simulink model "Project2"  (R2024b)
settings: Solver=VariableStepAuto  StartTime=0.0  StopTime=4  RelTol=1e-3
values from neighbouring files (symbols this model uses):
  Cl = 2000e-6    (= 0.002)    [ScriptFile.m]
  ka = Vdcref / 2    (= 350)    [ScriptFile.m]
  kii = 2 * pi * fbwi * Rl / ka    (= 0.0538558740615)    [ScriptFile.m]
  kiw = Vq / Vdcref    [ScriptFile.m]
  kpi = 2 * pi * fbwi * Ll / ka    (= 0.134639685154)    [ScriptFile.m]
  kpw = 2 * Cl / (kiw * a_l * tau1l)    [ScriptFile.m]
  Ll = 5e-3    (= 0.005)    [ScriptFile.m]
  Rbat = (Vdcref / Pdc) * (Vbat - Vdcref)    (= 7)    [ScriptFile.m]
  Rl = 0.002    [ScriptFile.m]
  tau_fl = 1 / (2 * pi * 100)    (= 0.00159154943092)    [ScriptFile.m]
  Vdcref = 700    [ScriptFile.m]
libraries: spsVoltageMeasurementLib x7, spsIGBTDiodeLib x6, spsSeriesRLCBranchLib x4, spsCurrentMeasurementLib x3, simulink x3, spsThreePhaseSeriesRLCBranchLib x2, spsBreakerLib x1, spsControlledVoltageSourceLib x1, spsTriangleGeneratorLib x1, spsThreePhaseBreakerLib x1, spsThreePhaseSourceLib x1, sps_lib x1
settings Model: Creator=SSP Family  LastModifiedBy=PREKSHA

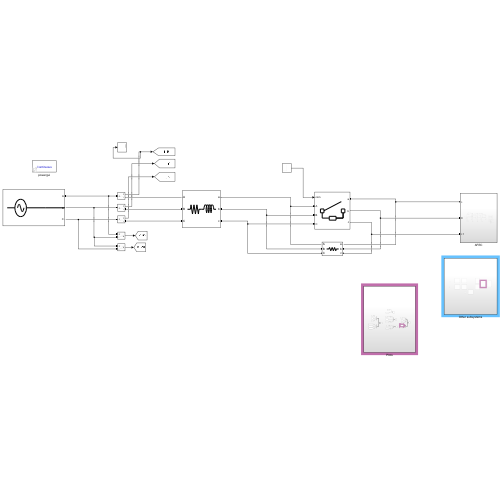
[thumbnail: Simulink's stored preview of the top-level diagram]
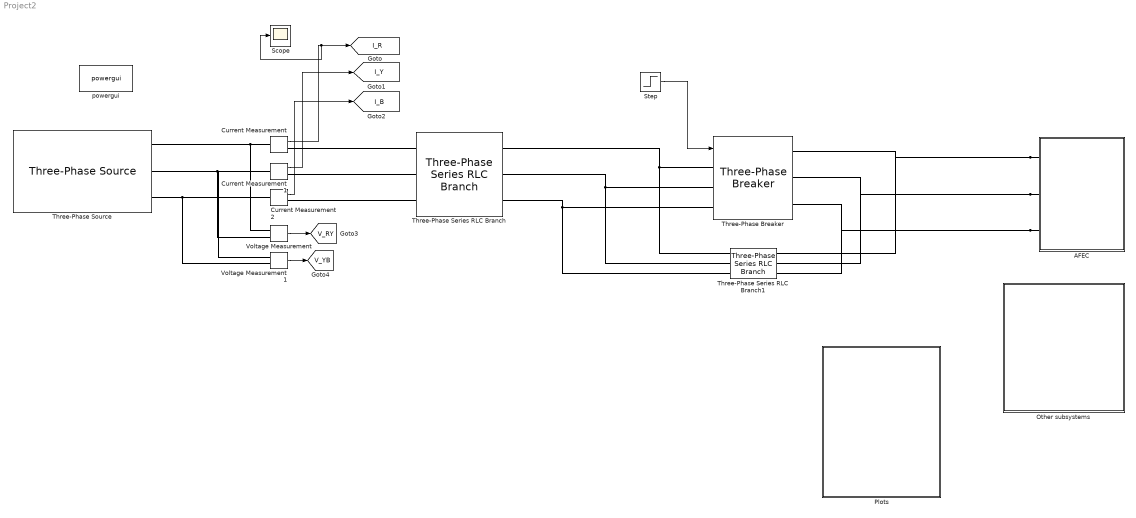
== system Project2 ==
  AFEC : Subsystem
  Current Measurement : spsCurrentMeasurementLib/Current Measurement  PhasorSimulation=off  OutputType=Complex  PSBequivalent=0
  Current Measurement1 : spsCurrentMeasurementLib/Current Measurement  PhasorSimulation=off  OutputType=Complex  PSBequivalent=0
  Current Measurement2 : spsCurrentMeasurementLib/Current Measurement  PhasorSimulation=off  OutputType=Complex  PSBequivalent=0
  Other subsystems : Subsystem
  Plots : Subsystem
  Scope : Scope
  Step : Step  Time=0.4  SampleTime=0
  Three-Phase Series RLC Branch : spsThreePhaseSeriesRLCBranchLib/Three-Phase Series RLC Branch  LConnTagsString=A|B|C  RConnTagsString=A|B|C  BranchType=RL  Resistance=Rl  Inductance=Ll  Capacitance=1e-6  Measurements=None
  Three-Phase Series RLC Branch1 : spsThreePhaseSeriesRLCBranchLib/Three-Phase Series RLC Branch  LConnTagsString=A|B|C  RConnTagsString=A|B|C  BranchType=R  Resistance=100  Inductance=1e-3  Capacitance=1e-6  Measurements=None
  Three-Phase Breaker : spsThreePhaseBreakerLib/Three-Phase Breaker  InitialState=open  SwitchA=on  SwitchB=on  SwitchC=on  SwitchTimes="[1/60  5/60]"  External=on  BreakerResistance=0.01  SnubberResistance=1e6  SnubberCapacitance=inf  Measurements=None
  Three-Phase Source : spsThreePhaseSourceLib/Three-Phase Source  InternalConnection=Y  VoltagePhases=off  Voltage=400/sqrt(3)  PhaseAngle=0  Voltage_phases=[25e3 25e3 25e3]/sqrt(3)  PhaseAngles_phases=[0 -120 +120]  Frequency=50  NonIdealSource=off  SpecifyImpedance=off  Resistance=0  Inductance=0  ShortCircuitLevel=100e6  BaseVoltage=25e3  XRratio=7  BusType=swing  Pref=10e3  Qref=0  Prefabc=[10e3, 10e3, 10e3]  Qrefabc=[0, 0, 0]  Qmin=-inf  Qmax=inf
  Voltage Measurement : spsVoltageMeasurementLib/Voltage Measurement  PhasorSimulation=off  OutputType=Complex  PSBequivalent=0
  Voltage Measurement1 : spsVoltageMeasurementLib/Voltage Measurement  PhasorSimulation=off  OutputType=Complex  PSBequivalent=0
  powergui : sps_lib/powergui  Priority=1  SimulationMode=Continuous  SampleTime=50e-6  frequency=60  Iterations=50  frequencyindice=50  Pbase=100e6  ErrMax=1e-4  UnitsV=kV  UnitsW=MW  buscounter=0  FunctionMessages=off  echomessages=off  EnableUseOfTLC=off  CurrentSourceSwitches=off  DisableSnubberDevices=off  DisableRonSwitches=off  DisableVfSwitches=off  DisplayEquations=off  AutomaticDiscreteSolvers=off  SolverType=Tustin/Backward Euler (TBE)  Interpol=off  ExternalGateDelay=off  methode=off  Ts=100  x0status=blocks  SPID=on  SwTol=0  HookPort=off  NonlinearTolerance=1e-4  nMaxIteration=100  ContinueOnMaxIteration=off  RestoreLinks=warning  ResistiveCurrentMeasurement=off  Frange=[0:2:500]  Ylog=off  Xlog=on  ShowGrid=off  save=off  variable=ZData  structure=0  ZoomFFT=off  StartTime=0.0  cycles=1  DisplayStyle=1  fundamental=60  FreqAxis=off  MaxFrequency=1000  frequencyindicesteady=1  RmsSteady=1  display=off
  tag scope: I_B=global, I_R=global, I_Y=global, V_RY=global, V_YB=global
  wires:
  Voltage Measurement/1 -> [V_RY]
  Voltage Measurement1/1 -> [V_YB]
  Step/1 -> Three-Phase Breaker/1
  Current Measurement/1 -> Scope/1, [I_R]
  Current Measurement1/1 -> [I_Y]
  Current Measurement2/1 -> [I_B]
  connections:
  Current Measurement/LConn1 -- Voltage Measurement/LConn1 -- Three-Phase Source/RConn1
  Current Measurement1/LConn1 -- Voltage Measurement1/LConn1 -- Voltage Measurement/LConn2 -- Three-Phase Source/RConn2
  Three-Phase Source/RConn3 -- Voltage Measurement1/LConn2 -- Current Measurement2/LConn1
  Current Measurement/RConn1 -- Three-Phase Series RLC Branch/LConn1
  Current Measurement1/RConn1 -- Three-Phase Series RLC Branch/LConn2
  Current Measurement2/RConn1 -- Three-Phase Series RLC Branch/LConn3
  Three-Phase Series RLC Branch1/LConn2 -- Three-Phase Series RLC Branch/RConn2 -- Three-Phase Breaker/LConn2
  Three-Phase Series RLC Branch1/LConn1 -- Three-Phase Series RLC Branch/RConn1 -- Three-Phase Breaker/LConn1
  AFEC/LConn1 -- Three-Phase Breaker/RConn1 -- Three-Phase Series RLC Branch1/RConn1
  Three-Phase Series RLC Branch1/LConn3 -- Three-Phase Series RLC Branch/RConn3 -- Three-Phase Breaker/LConn3
  AFEC/LConn3 -- Three-Phase Breaker/RConn3 -- Three-Phase Series RLC Branch1/RConn3
  AFEC/LConn2 -- Three-Phase Breaker/RConn2 -- Three-Phase Series RLC Branch1/RConn2

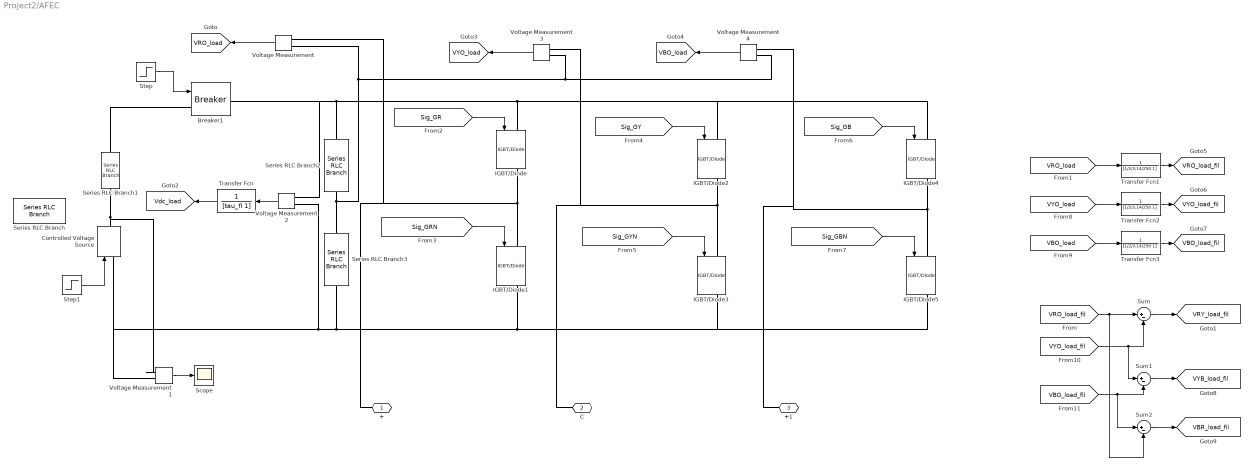
== system Project2/AFEC ==
  Breaker1 : spsBreakerLib/Breaker  InitialState=0  SwitchingTimes="[1/60  5/60]"  External=on  BreakerResistance=0.01  SnubberResistance=1e6  SnubberCapacitance=inf  Measurements=None  MoreParameters=on  NoBreakLoop=off
  Controlled Voltage Source : spsControlledVoltageSourceLib/Controlled Voltage Source  Initialize=on  Source_Type=DC  Amplitude=800  Phase=0  Frequency=0  Measurements=None
  IGBT/Diode{,1..5} (6 alike) : spsIGBTDiodeLib/IGBT//Diode  Ron=1e-3  Rs=1e5  Cs=inf  Measurements=on
  Scope : Scope
  Series RLC Branch : spsSeriesRLCBranchLib/Series RLC Branch  LConnTagsString=__new0  RConnTagsString=__new0  BranchType=R  Resistance=50  Inductance=1e-3  SetiL0=off  InitialCurrent=0  Capacitance=1e-6  Setx0=off  InitialVoltage=0  Measurements=None
  Series RLC Branch1 : spsSeriesRLCBranchLib/Series RLC Branch  LConnTagsString=__new0  RConnTagsString=__new0  BranchType=R  Resistance=Rbat  Inductance=1e-3  SetiL0=off  InitialCurrent=0  Capacitance=1e-6  Setx0=off  InitialVoltage=0  Measurements=None
  Series RLC Branch2 : spsSeriesRLCBranchLib/Series RLC Branch  LConnTagsString=__new0  RConnTagsString=__new0  BranchType=C  Resistance=1  Inductance=1e-3  SetiL0=off  InitialCurrent=0  Capacitance=Cl  Setx0=off  InitialVoltage=0  Measurements=None
  Series RLC Branch3 : spsSeriesRLCBranchLib/Series RLC Branch  LConnTagsString=__new0  RConnTagsString=__new0  BranchType=C  Resistance=1  Inductance=1e-3  SetiL0=off  InitialCurrent=0  Capacitance=Cl  Setx0=off  InitialVoltage=0  Measurements=None
  Step : Step  Time=3  SampleTime=0
  Step1 : Step  Time=2  Before=1  After=0  SampleTime=0
  Sum : Sum  Inputs=|+-
  Sum1 : Sum  Inputs=|+-
  Sum2 : Sum  Inputs=|+-
  Transfer Fcn : TransferFcn  Denominator=[tau_fl 1]
  Transfer Fcn1 : TransferFcn  Denominator=[1/2/3.14/250 1]
  Transfer Fcn2 : TransferFcn  Denominator=[1/2/3.14/250 1]
  Transfer Fcn3 : TransferFcn  Denominator=[1/2/3.14/250 1]
  Voltage Measurement{,1..4} (5 alike) : spsVoltageMeasurementLib/Voltage Measurement  PhasorSimulation=off  OutputType=Complex  PSBequivalent=0
  + : PMIOPort  Side=Left
  C : PMIOPort  Port=2  Side=Left
  +1 : PMIOPort  Port=3  Side=Left
  tag scope: VBO_load=global, VBO_load_fil=global, VBR_load_fil=global, VRO_load=global, VRO_load_fil=global, VRY_load_fil=global, VYB_load_fil=global, VYO_load=global, VYO_load_fil=global, Vdc_load=global
  wires:
  Voltage Measurement4/1 -> [VBO_load]
  [Sig_GBN] -> IGBT/Diode5/1
  Voltage Measurement3/1 -> [VYO_load]
  Transfer Fcn/1 -> [Vdc_load]
  [Sig_GB] -> IGBT/Diode4/1
  Voltage Measurement/1 -> [VRO_load]
  [Sig_GY] -> IGBT/Diode2/1
  Voltage Measurement2/1 -> Transfer Fcn/1
  [Sig_GRN] -> IGBT/Diode1/1
  [Sig_GYN] -> IGBT/Diode3/1
  [Sig_GR] -> IGBT/Diode/1
  [VBO_load] -> Transfer Fcn3/1
  Transfer Fcn2/1 -> [VYO_load_fil]
  [VRO_load] -> Transfer Fcn1/1
  Transfer Fcn3/1 -> [VBO_load_fil]
  Transfer Fcn1/1 -> [VRO_load_fil]
  [VYO_load] -> Transfer Fcn2/1
  [VRO_load_fil] -> Sum2/2, Sum/1
  [VYO_load_fil] -> Sum1/1, Sum/2
  [VBO_load_fil] -> Sum2/1, Sum1/2
  Sum/1 -> [VRY_load_fil]
  Sum1/1 -> [VYB_load_fil]
  Sum2/1 -> [VBR_load_fil]
  Step/1 -> Breaker1/1
  Step1/1 -> Controlled Voltage Source/1
  Voltage Measurement1/1 -> Scope/1
  connections:
  IGBT/Diode2/LConn1 -- IGBT/Diode4/LConn1 -- IGBT/Diode/LConn1 -- Breaker1/RConn1 -- Voltage Measurement2/LConn1 -- Series RLC Branch2/LConn1
  IGBT/Diode4/RConn1 -- Voltage Measurement4/LConn1 -- +1/RConn1 -- IGBT/Diode5/LConn1
  IGBT/Diode/RConn1 -- Voltage Measurement/LConn1 -- +/RConn1 -- IGBT/Diode1/LConn1
  Series RLC Branch3/RConn1 -- IGBT/Diode3/RConn1 -- IGBT/Diode5/RConn1 -- IGBT/Diode1/RConn1 -- Controlled Voltage Source/LConn1 -- Voltage Measurement1/LConn2 -- Voltage Measurement2/LConn2
  IGBT/Diode2/RConn1 -- IGBT/Diode3/LConn1 -- Voltage Measurement3/LConn1 -- C/RConn1
  Voltage Measurement3/LConn2 -- Voltage Measurement4/LConn2 -- Voltage Measurement/LConn2 -- Series RLC Branch2/RConn1 -- Series RLC Branch3/LConn1
  Controlled Voltage Source/RConn1 -- Series RLC Branch1/LConn1 -- Voltage Measurement1/LConn1
  Series RLC Branch1/RConn1 -- Breaker1/LConn1

== system Project2/Other subsystems ==
  FF compensation : Subsystem
  Gate sig generation : Subsystem
  I_Alpha-Beta to I_dq : Subsystem
  I_RYB to I_Alpha-Beta : Subsystem
  PI for PLL : Subsystem
  Phase locked loop : Subsystem  Commented=on
  Subsystem : Subsystem  Commented=on
  Subsystem1 : Subsystem  Commented=on
  V_Alpha-Beta to V_dq : Subsystem
  V_RYB to V_Alpha-Beta : Subsystem
  d-axis current controller : Subsystem
  dc link voltage controller + q-axis current controller : Subsystem

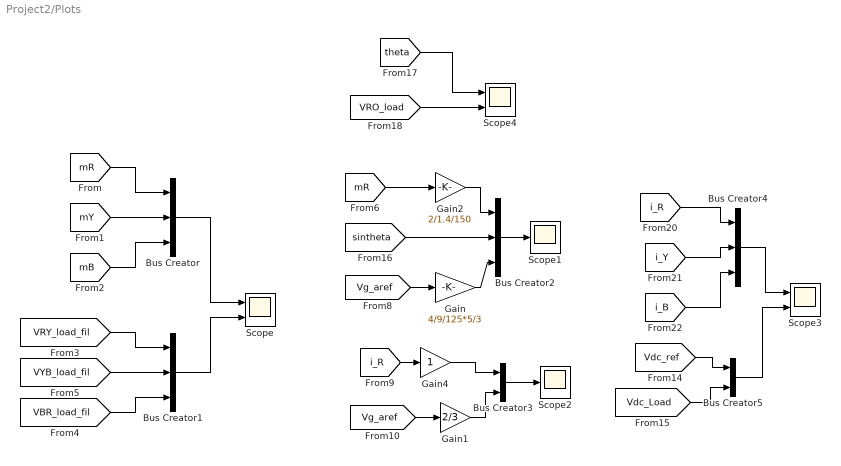
== system Project2/Plots ==
  Bus Creator{,1..2,4} (4 alike) : BusCreator  Inputs=3
  Bus Creator3 : BusCreator  Inputs=2
  Bus Creator5 : BusCreator  Inputs=2
  Gain : Gain  Gain=4/9/125*5/3
  Gain1 : Gain  Gain=2/3
  Gain2 : Gain  Gain=2/1.4/150
  Gain4 : Gain
  Scope : Scope  NumInputPorts=2
  Scope1 : Scope
  Scope2 : Scope
  Scope3 : Scope  NumInputPorts=2
  Scope4 : Scope  NumInputPorts=2
  wires:
  [mB] -> Bus Creator/3
  [VYB_load_fil] -> Bus Creator1/2
  Bus Creator/1 -> Scope/1
  Bus Creator3/1 -> Scope2/1
  [mY] -> Bus Creator/2
  Gain/1 -> Bus Creator2/3
  [Vg_aref] -> Gain/1
  [mR] -> Bus Creator/1
  Gain1/1 -> Bus Creator3/2
  [Vg_aref] -> Gain1/1
  [i_R] -> Gain4/1
  Bus Creator2/1 -> Scope1/1
  Bus Creator1/1 -> Scope/2
  [VBR_load_fil] -> Bus Creator1/3
  [VRY_load_fil] -> Bus Creator1/1
  Gain2/1 -> Bus Creator2/1
  [sintheta] -> Bus Creator2/2
  [mR] -> Gain2/1
  [theta] -> Scope4/1
  [VRO_load] -> Scope4/2
  Gain4/1 -> Bus Creator3/1
  [i_R] -> Bus Creator4/1
  [Vdc_Load] -> Bus Creator5/2
  [i_Y] -> Bus Creator4/2
  [Vdc_ref] -> Bus Creator5/1
  [i_B] -> Bus Creator4/3
  Bus Creator4/1 -> Scope3/1
  Bus Creator5/1 -> Scope3/2

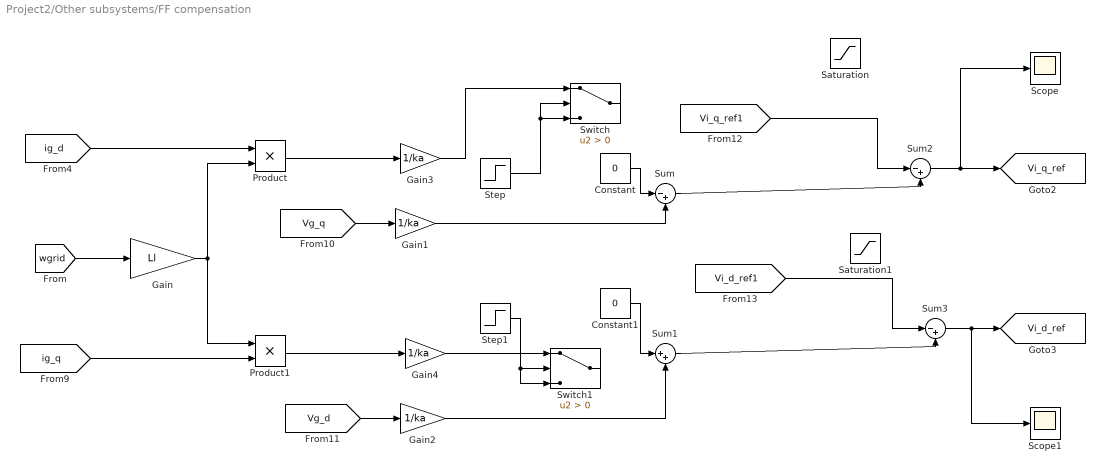
== system Project2/Other subsystems/FF compensation ==
  Constant : Constant  Value=0
  Constant1 : Constant  Value=0
  Gain : Gain  Gain=Ll
  Gain{1..4} (4 alike) : Gain  Gain=1/ka
  Product : Product
  Product1 : Product
  Saturation : Saturate  UpperLimit=1  LowerLimit=-1
  Saturation1 : Saturate  UpperLimit=1  LowerLimit=-1
  Scope : Scope
  Scope1 : Scope
  Step : Step  Time=2.5  SampleTime=0
  Step1 : Step  Time=2.5  SampleTime=0
  Sum : Sum  Inputs=|-+
  Sum1 : Sum  Inputs=|++
  Sum2 : Sum  Inputs=|-+
  Sum3 : Sum  Inputs=|-+
  Switch : Switch  Criteria=u2 > Threshold  SaturateOnIntegerOverflow=off  InputSameDT=off
  Switch1 : Switch  Criteria=u2 > Threshold  SaturateOnIntegerOverflow=off  InputSameDT=off
  tag scope: Vi_d_ref=global, Vi_q_ref=global
  wires:
  Sum3/1 -> Scope1/1, [Vi_d_ref]
  Gain2/1 -> Sum1/2
  [Vg_d] -> Gain2/1
  Step/1 -> Switch/3, Switch/2
  Sum/1 -> Sum2/2
  Gain/1 -> Product1/1, Product/2
  Gain1/1 -> Sum/2
  [Vi_q_ref1] -> Sum2/1
  Sum2/1 -> Scope/1, [Vi_q_ref]
  [ig_d] -> Product/1
  [Vi_d_ref1] -> Sum3/1
  [Vg_q] -> Gain1/1
  Sum1/1 -> Sum3/2
  Gain3/1 -> Switch/1
  Product/1 -> Gain3/1
  Product1/1 -> Gain4/1
  [wgrid] -> Gain/1
  [ig_q] -> Product1/2
  Step1/1 -> Switch1/3, Switch1/2
  Gain4/1 -> Switch1/1
  Constant/1 -> Sum/1
  Constant1/1 -> Sum1/1

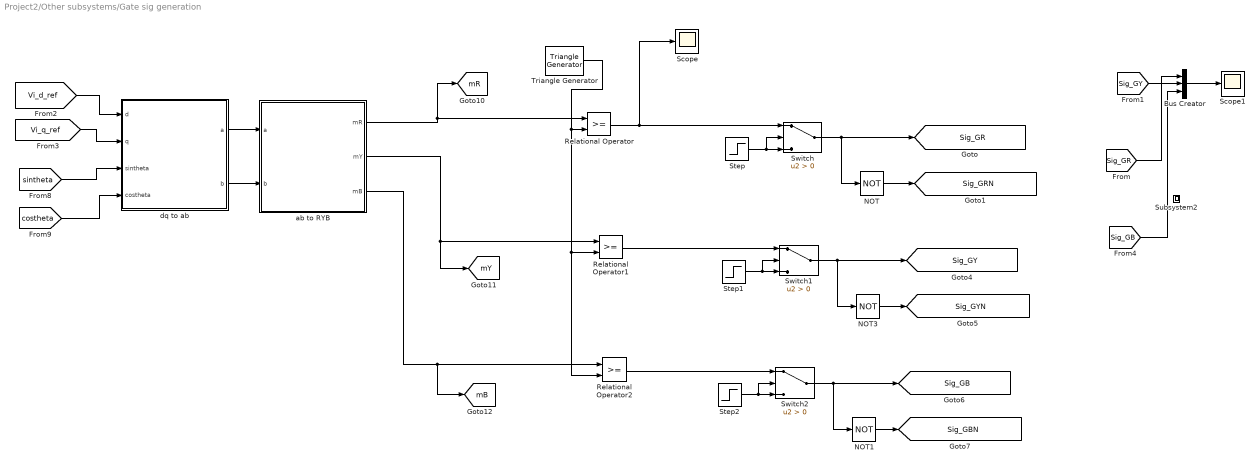
== system Project2/Other subsystems/Gate sig generation ==
  Bus Creator : BusCreator  Inputs=3
  NOT : Logic  Operator=NOT  IconShape=distinctive  AllPortsSameDT=off  OutDataTypeStr=boolean
  NOT1 : Logic  Operator=NOT  IconShape=distinctive  AllPortsSameDT=off  OutDataTypeStr=boolean
  NOT3 : Logic  Operator=NOT  IconShape=distinctive  AllPortsSameDT=off  OutDataTypeStr=boolean
  Relational Operator : RelationalOperator  OutDataTypeStr=boolean  RndMeth=Simplest  InputSameDT=off
  Relational Operator1 : RelationalOperator  OutDataTypeStr=boolean  RndMeth=Simplest  InputSameDT=off
  Relational Operator2 : RelationalOperator  OutDataTypeStr=boolean  RndMeth=Simplest  InputSameDT=off
  Scope : Scope
  Scope1 : Scope
  Step : Step  SampleTime=0
  Step1 : Step  SampleTime=0
  Step2 : Step  SampleTime=0
  Subsystem2 : Subsystem
  Switch : Switch  Criteria=u2 > Threshold  SaturateOnIntegerOverflow=off  InputSameDT=off
  Switch1 : Switch  Criteria=u2 > Threshold  SaturateOnIntegerOverflow=off  InputSameDT=off
  Switch2 : Switch  Criteria=u2 > Threshold  SaturateOnIntegerOverflow=off  InputSameDT=off
  Triangle Generator : spsTriangleGeneratorLib/Triangle Generator  Freq=fsw  Phase=90  Ts=0
  ab to RYB : MATLAB Function  TreatAsAtomicUnit=on
  dq to ab : MATLAB Function  TreatAsAtomicUnit=on
  tag scope: Sig_GB=global, Sig_GBN=global, Sig_GR=global, Sig_GRN=global, Sig_GY=global, Sig_GYN=global, mB=global, mR=global, mY=global
  wires:
  dq to ab/1(a) -> ab to RYB/1(a)
  [Vi_q_ref] -> dq to ab/2(q)
  ab to RYB/2(mY) -> [mY], Relational Operator1/1
  Triangle Generator/1 -> Relational Operator2/2, Relational Operator1/2, Relational Operator/2
  Relational Operator/1 -> Scope/1, Switch/1
  [sintheta] -> dq to ab/3(sintheta)
  [costheta] -> dq to ab/4(costheta)
  dq to ab/2(b) -> ab to RYB/2(b)
  [Vi_d_ref] -> dq to ab/1(d)
  ab to RYB/1(mR) -> Relational Operator/1, [mR]
  ab to RYB/3(mB) -> Relational Operator2/1, [mB]
  Step/1 -> Switch/2, Switch/3
  Switch/1 -> NOT/1, [Sig_GR]
  NOT/1 -> [Sig_GRN]
  NOT3/1 -> [Sig_GYN]
  Step1/1 -> Switch1/2, Switch1/3
  Relational Operator1/1 -> Switch1/1
  Switch1/1 -> [Sig_GY], NOT3/1
  Relational Operator2/1 -> Switch2/1
  NOT1/1 -> [Sig_GBN]
  Step2/1 -> Switch2/2, Switch2/3
  Switch2/1 -> [Sig_GB], NOT1/1
  [Sig_GR] -> Bus Creator/1
  [Sig_GY] -> Bus Creator/2
  [Sig_GB] -> Bus Creator/3
  Bus Creator/1 -> Scope1/1

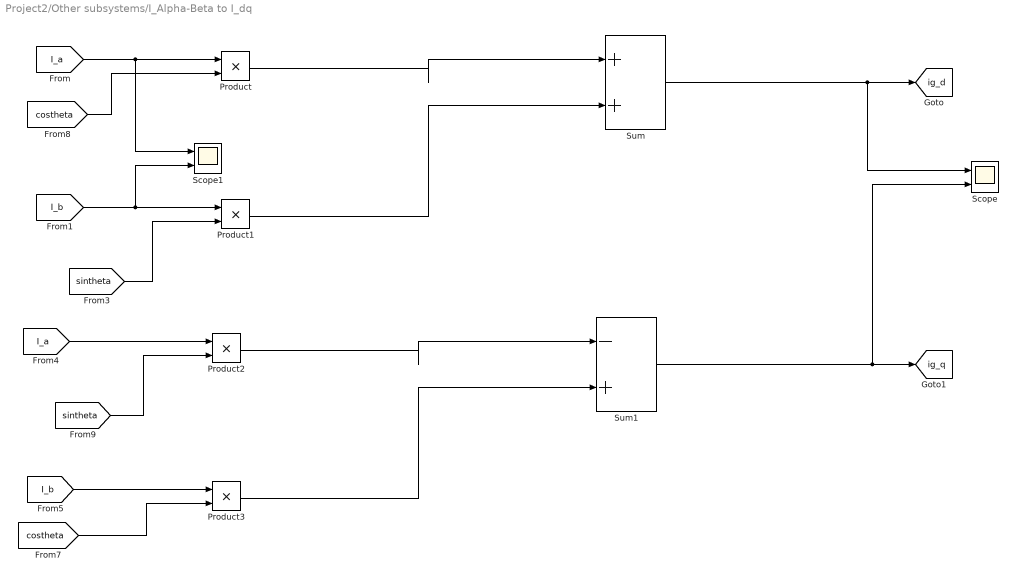
== system Project2/Other subsystems/I_Alpha-Beta to I_dq ==
  Product{,1..3} (4 alike) : Product
  Scope : Scope  NumInputPorts=2
  Scope1 : Scope  NumInputPorts=2
  Sum : Sum  Inputs=|++
  Sum1 : Sum  Inputs=|-+
  tag scope: ig_d=global, ig_q=global
  wires:
  Product1/1 -> Sum/2
  [I_a] -> Product2/1
  [I_b] -> Product3/1
  [sintheta] -> Product1/2
  [sintheta] -> Product2/2
  Product2/1 -> Sum1/1
  Product/1 -> Sum/1
  Product3/1 -> Sum1/2
  Sum1/1 -> [ig_q], Scope/2
  Sum/1 -> Scope/1, [ig_d]
  [I_a] -> Scope1/1, Product/1
  [I_b] -> Product1/1, Scope1/2
  [costheta] -> Product/2
  [costheta] -> Product3/2

== system Project2/Other subsystems/I_RYB to I_Alpha-Beta ==
  Gain : Gain  Gain=2/3
  Gain1 : Gain
  Gain2 : Gain  Gain=-1/2
  Gain3 : Gain  Gain=-1/2
  Gain4 : Gain  Gain=2/3
  Gain5 : Gain  Gain=0
  Gain6 : Gain  Gain=sqrt(3)/2
  Gain7 : Gain  Gain=-sqrt(3)/2
  Scope1 : Scope  NumInputPorts=2
  Sine Wave : Sin  Amplitude=200*sqrt(6)  Frequency=100*pi  Phase=pi/6  SampleTime=0
  Sine Wave1 : Sin  Amplitude=200*sqrt(6)  Frequency=100*pi  Phase=-pi/2  SampleTime=0
  Sum : Sum  Inputs=|+++
  Sum1 : Sum  Inputs=|+++
  tag scope: I_a=global, I_b=global
  wires:
  Sum/1 -> Gain/1
  Gain1/1 -> Sum/1
  Gain2/1 -> Sum/2
  Gain3/1 -> Sum/3
  Gain/1 -> Scope1/1, [I_a]
  Gain4/1 -> Scope1/2, [I_b]
  Gain7/1 -> Sum1/3
  Gain6/1 -> Sum1/2
  Gain5/1 -> Sum1/1
  Sum1/1 -> Gain4/1
  [I_R] -> Gain5/1, Gain1/1
  [I_Y] -> Gain6/1, Gain2/1
  [I_B] -> Gain7/1, Gain3/1

== system Project2/Other subsystems/PI for PLL ==
  Center Frequency : Constant  Value=2*pi*50
  Constant : Constant  Value=2*pi
  Gain : Gain
  Gain1 : Gain
  Integrator : Integrator  LimitOutput=on  UpperSaturationLimit=2*pi*50  LowerSaturationLimit=-2*pi*50
  Integrator1 : Integrator
  Mod : Math  Operator=mod
  Saturation : Saturate  UpperLimit=2*pi*50  LowerLimit=-2*pi*50
  Scope : Scope
  Step : Step  Time=.3  SampleTime=0
  Sum : Sum  Inputs=|-+
  Sum1 : Sum  Inputs=|++
  Sum2 : Sum  Inputs=|++
  Switch : Switch  Criteria=u2 > Threshold  SaturateOnIntegerOverflow=off  InputSameDT=off
  V_d_ref : Constant  Value=0
  tag scope: theta=global, wgrid=global
  wires:
  [Vg_d] -> Sum/1
  V_d_ref/1 -> Sum/2
  Gain1/1 -> Integrator/1
  Gain/1 -> Sum1/1
  Integrator/1 -> Sum1/2
  Sum1/1 -> Saturation/1
  Center Frequency/1 -> Sum2/2
  Sum2/1 -> [wgrid], Integrator1/1
  Integrator1/1 -> Mod/1
  Constant/1 -> Mod/2
  Mod/1 -> Scope/1, [theta]
  Saturation/1 -> Sum2/1
  Sum/1 -> Switch/1
  Step/1 -> Switch/3, Switch/2
  Switch/1 -> Gain/1, Gain1/1

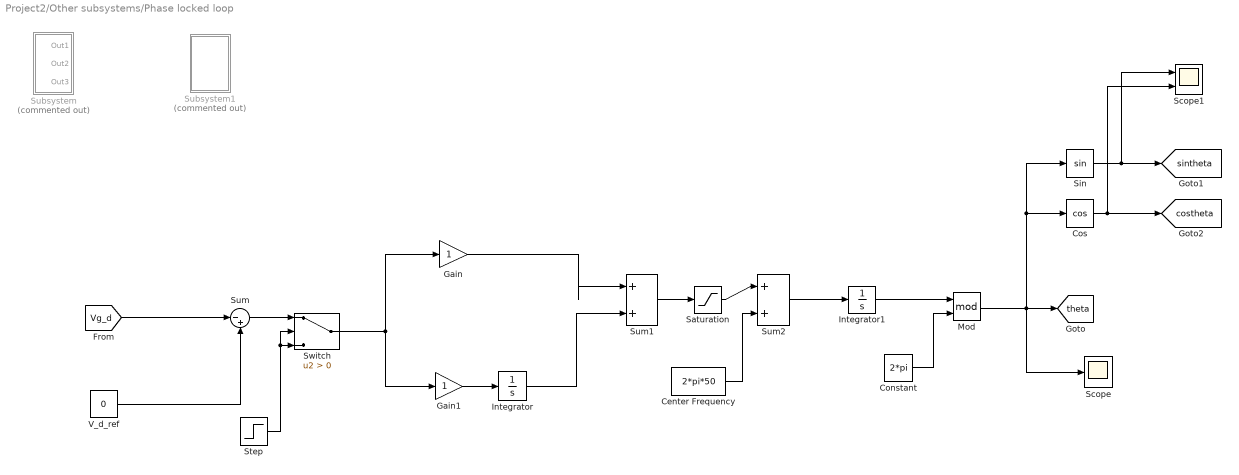
== system Project2/Other subsystems/Phase locked loop ==
  Center Frequency : Constant  Value=2*pi*50
  Constant : Constant  Value=2*pi
  Cos : Trigonometry  Operator=cos
  Gain : Gain
  Gain1 : Gain
  Integrator : Integrator  LimitOutput=on  UpperSaturationLimit=2*pi*50  LowerSaturationLimit=-2*pi*50
  Integrator1 : Integrator
  Mod : Math  Operator=mod
  Saturation : Saturate  UpperLimit=2*pi*50  LowerLimit=-2*pi*50
  Scope : Scope
  Scope1 : Scope  NumInputPorts=2
  Sin : Trigonometry
  Step : Step  Time=0  SampleTime=0
  Subsystem : Subsystem  Commented=on
  Subsystem1 : Subsystem  Commented=on
  Sum : Sum  Inputs=|-+
  Sum1 : Sum  Inputs=|++
  Sum2 : Sum  Inputs=|++
  Switch : Switch  Criteria=u2 > Threshold  SaturateOnIntegerOverflow=off  InputSameDT=off
  V_d_ref : Constant  Value=0
  tag scope: costheta=global, sintheta=global, theta=global
  wires:
  Center Frequency/1 -> Sum2/2
  Mod/1 -> Sin/1, Cos/1, Scope/1, [theta]
  Gain1/1 -> Integrator/1
  Saturation/1 -> Sum2/1
  Sum1/1 -> Saturation/1
  Constant/1 -> Mod/2
  Gain/1 -> Sum1/1
  Integrator1/1 -> Mod/1
  Sum2/1 -> Integrator1/1
  Integrator/1 -> Sum1/2
  V_d_ref/1 -> Sum/2
  [Vg_d] -> Sum/1
  Sin/1 -> Scope1/1, [sintheta]
  Sum/1 -> Switch/1
  Step/1 -> Switch/3, Switch/2
  Switch/1 -> Gain/1, Gain1/1
  Cos/1 -> [costheta], Scope1/2

== system Project2/Other subsystems/Subsystem ==
  ry : Inport
  yb : Inport  Port=2
  ab to dq (1) : MATLAB Function  TreatAsAtomicUnit=on
  ry,yb to ab : MATLAB Function  TreatAsAtomicUnit=on
  tag scope: Vg_a_ref=global, Vg_b_ref=global, Vg_d=global, Vg_q=global
  wires:
  ry,yb to ab/1(a) -> [Vg_a_ref], ab to dq (1)/1(a)
  ry,yb to ab/2(b) -> [Vg_b_ref], ab to dq (1)/2(b)
  [sintheta] -> ab to dq (1)/3(sintheta)
  ab to dq (1)/1(d) -> [Vg_d]
  yb/1 -> ry,yb to ab/2(yb)
  ab to dq (1)/2(q) -> [Vg_q]
  ry/1 -> ry,yb to ab/1(ry)
  [costheta] -> ab to dq (1)/4(costheta)

== system Project2/Other subsystems/Subsystem1 ==
  ab to dq : MATLAB Function  TreatAsAtomicUnit=on
  ryb to ab : MATLAB Function  TreatAsAtomicUnit=on
  tag scope: ig_d=global, ig_q=global
  wires:
  ab to dq/1(d) -> [ig_d]
  [sintheta] -> ab to dq/3(sintheta)
  [I_Y] -> ryb to ab/2(y)
  [I_R] -> ryb to ab/1(r)
  ryb to ab/1(a) -> ab to dq/1(a)
  ab to dq/2(q) -> [ig_q]
  ryb to ab/2(b) -> ab to dq/2(b)
  [costheta] -> ab to dq/4(costheta)
  [I_B] -> ryb to ab/3("b ")

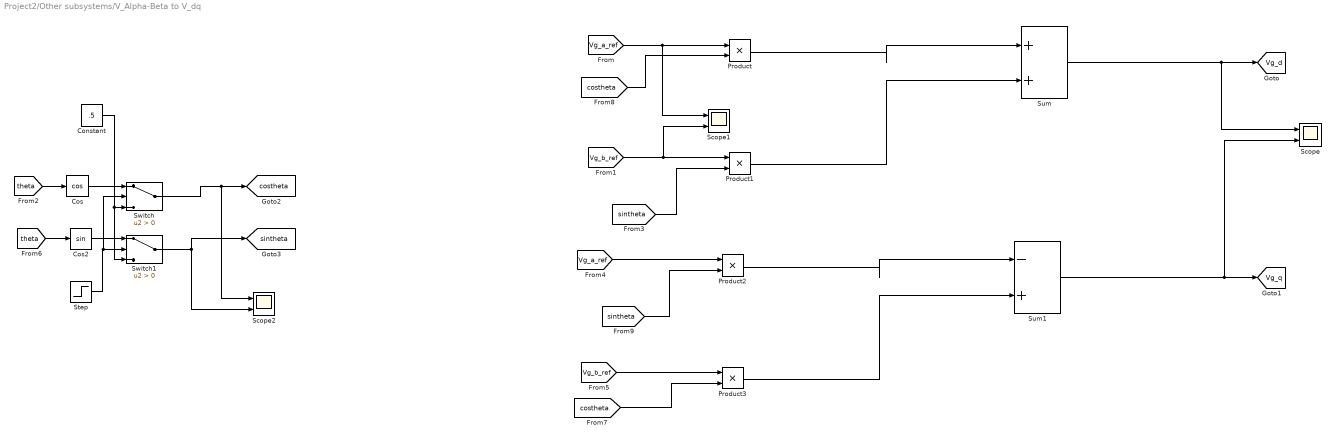
== system Project2/Other subsystems/V_Alpha-Beta to V_dq ==
  Constant : Constant  Value=.5
  Cos : Trigonometry  Operator=cos
  Cos2 : Trigonometry
  Product{,1..3} (4 alike) : Product
  Scope : Scope  NumInputPorts=2
  Scope1 : Scope  NumInputPorts=2
  Scope2 : Scope  NumInputPorts=2
  Step : Step  Time=.3  SampleTime=0
  Sum : Sum  Inputs=|++
  Sum1 : Sum  Inputs=|-+
  Switch : Switch  Criteria=u2 > Threshold  SaturateOnIntegerOverflow=off  InputSameDT=off
  Switch1 : Switch  Criteria=u2 > Threshold  SaturateOnIntegerOverflow=off  InputSameDT=off
  tag scope: Vg_d=global, Vg_q=global, costheta=global, sintheta=global
  wires:
  Product1/1 -> Sum/2
  [Vg_a_ref] -> Product2/1
  [Vg_b_ref] -> Product3/1
  [sintheta] -> Product1/2
  [sintheta] -> Product2/2
  Product2/1 -> Sum1/1
  Product/1 -> Sum/1
  Product3/1 -> Sum1/2
  Sum1/1 -> [Vg_q], Scope/2
  Sum/1 -> Scope/1, [Vg_d]
  [Vg_a_ref] -> Scope1/1, Product/1
  [Vg_b_ref] -> Product1/1, Scope1/2
  [theta] -> Cos/1
  [costheta] -> Product/2
  [costheta] -> Product3/2
  [theta] -> Cos2/1
  Cos/1 -> Switch/1
  Switch/1 -> Scope2/1, [costheta]
  Cos2/1 -> Switch1/1
  Constant/1 -> Switch1/3, Switch/3
  Step/1 -> Switch/2, Switch1/2
  Switch1/1 -> [sintheta], Scope2/2

== system Project2/Other subsystems/V_RYB to V_Alpha-Beta ==
  Gain : Gain  Gain=2/3
  Gain1 : Gain
  Gain2 : Gain  Gain=-1/2
  Gain3 : Gain  Gain=-1/2
  Gain4 : Gain  Gain=2/3
  Gain5 : Gain  Gain=0
  Gain6 : Gain  Gain=sqrt(3)/2
  Gain7 : Gain  Gain=-sqrt(3)/2
  MATLAB Function : MATLAB Function  TreatAsAtomicUnit=on
  Scope1 : Scope  NumInputPorts=2
  Sine Wave : Sin  Amplitude=200*sqrt(6)  Frequency=100*pi  Phase=pi/6  SampleTime=0
  Sine Wave1 : Sin  Amplitude=200*sqrt(6)  Frequency=100*pi  Phase=-pi/2  SampleTime=0
  Sum : Sum  Inputs=|+++
  Sum1 : Sum  Inputs=|+++
  tag scope: Vg_a_ref=global, Vg_b_ref=global
  wires:
  Sum/1 -> Gain/1
  Gain1/1 -> Sum/1
  Gain2/1 -> Sum/2
  Gain3/1 -> Sum/3
  Gain/1 -> Scope1/1, [Vg_a_ref]
  Gain4/1 -> Scope1/2, [Vg_b_ref]
  Gain7/1 -> Sum1/3
  Gain6/1 -> Sum1/2
  Gain5/1 -> Sum1/1
  Sum1/1 -> Gain4/1
  [V_YB] -> MATLAB Function/2(yb)
  [V_RY] -> MATLAB Function/1(ry)
  MATLAB Function/1(r) -> Gain5/1, Gain1/1
  MATLAB Function/2(y) -> Gain6/1, Gain2/1
  MATLAB Function/3(b) -> Gain7/1, Gain3/1

== system Project2/Other subsystems/d-axis current controller ==
  Bus Creator : BusCreator  Inputs=2
  Constant : Constant  Value=0
  Gain : Gain  Gain=kpi
  Gain1 : Gain  Gain=kii
  Integrator Limited : Integrator  LimitOutput=on  UpperSaturationLimit=1  LowerSaturationLimit=0
  Saturation : Saturate  UpperLimit=1  LowerLimit=-1
  Scope : Scope
  Scope1 : Scope
  Scope2 : Scope
  Step : Step  SampleTime=0
  Sum : Sum  Inputs=|+-
  Sum1 : Sum  Inputs=|++
  Switch : Switch  Criteria=u2 > Threshold  SaturateOnIntegerOverflow=off  InputSameDT=off
  tag scope: Vi_d_ref1=global
  wires:
  Constant/1 -> Sum/1, Bus Creator/1
  Gain1/1 -> Integrator Limited/1
  Bus Creator/1 -> Scope/1
  Switch/1 -> Gain/1, Gain1/1
  Integrator Limited/1 -> Sum1/2
  Sum1/1 -> Scope2/1, Scope1/1, [Vi_d_ref1]
  Sum/1 -> Switch/1
  Gain/1 -> Sum1/1
  Step/1 -> Switch/3, Switch/2
  [ig_d] -> Bus Creator/2, Sum/2

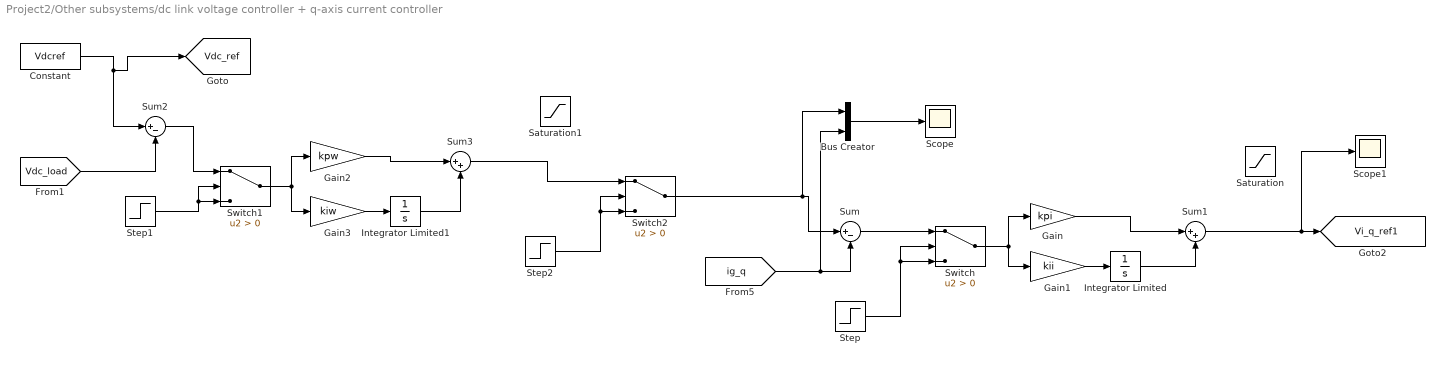
== system Project2/Other subsystems/dc link voltage controller + q-axis current controller ==
  Bus Creator : BusCreator  Inputs=2
  Constant : Constant  Value=Vdcref
  Gain : Gain  Gain=kpi
  Gain1 : Gain  Gain=kii
  Gain2 : Gain  Gain=kpw
  Gain3 : Gain  Gain=kiw
  Integrator Limited : Integrator  LimitOutput=on  UpperSaturationLimit=1.5  LowerSaturationLimit=-1.5
  Integrator Limited1 : Integrator  LimitOutput=on  UpperSaturationLimit=20  LowerSaturationLimit=-20
  Saturation : Saturate  UpperLimit=1  LowerLimit=-1
  Saturation1 : Saturate  UpperLimit=20  LowerLimit=-20
  Scope : Scope
  Scope1 : Scope
  Step : Step  SampleTime=0
  Step1 : Step  Time=2.5  SampleTime=0
  Step2 : Step  SampleTime=0
  Sum : Sum  Inputs=|+-
  Sum1 : Sum  Inputs=|++
  Sum2 : Sum  Inputs=|+-
  Sum3 : Sum  Inputs=|++
  Switch : Switch  Criteria=u2 > Threshold  SaturateOnIntegerOverflow=off  InputSameDT=off
  Switch1 : Switch  Criteria=u2 > Threshold  SaturateOnIntegerOverflow=off  InputSameDT=off
  Switch2 : Switch  Criteria=u2 > Threshold  SaturateOnIntegerOverflow=off  InputSameDT=off
  tag scope: Vdc_ref=global, Vi_q_ref1=global
  wires:
  Sum/1 -> Switch/1
  Switch2/1 -> Bus Creator/1, Sum/1
  Step/1 -> Switch/3, Switch/2
  Bus Creator/1 -> Scope/1
  Integrator Limited/1 -> Sum1/2
  [ig_q] -> Bus Creator/2, Sum/2
  Sum1/1 -> Scope1/1, [Vi_q_ref1]
  Switch/1 -> Gain/1, Gain1/1
  Gain/1 -> Sum1/1
  Gain1/1 -> Integrator Limited/1
  Sum2/1 -> Switch1/1
  Gain3/1 -> Integrator Limited1/1
  Gain2/1 -> Sum3/1
  Step1/1 -> Switch1/3, Switch1/2
  Step2/1 -> Switch2/3, Switch2/2
  Switch1/1 -> Gain3/1, Gain2/1
  [Vdc_load] -> Sum2/2
  Integrator Limited1/1 -> Sum3/2
  Constant/1 -> [Vdc_ref], Sum2/1
  Sum3/1 -> Switch2/1

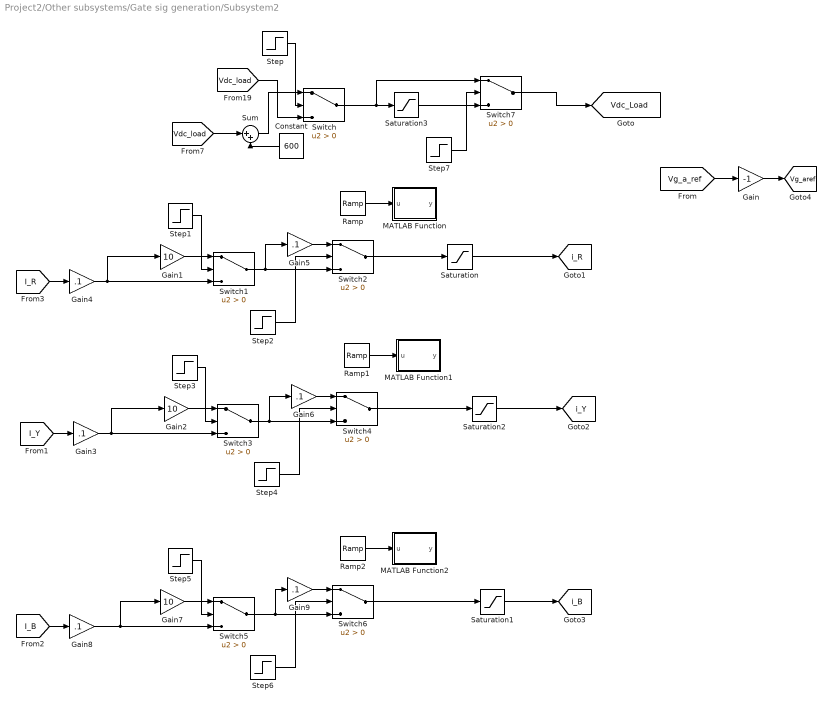
== system Project2/Other subsystems/Gate sig generation/Subsystem2 ==
  Constant : Constant  Value=600
  Gain : Gain  Gain=-1
  Gain1 : Gain  Gain=10
  Gain2 : Gain  Gain=10
  Gain{3..6,8..9} (6 alike) : Gain  Gain=.1
  Gain7 : Gain  Gain=10
  MATLAB Function : MATLAB Function  TreatAsAtomicUnit=on
  MATLAB Function1 : MATLAB Function  TreatAsAtomicUnit=on
  MATLAB Function2 : MATLAB Function  TreatAsAtomicUnit=on
  Ramp : simulink/Sources/Ramp  slope=1  start=3  InitialOutput=0
  Ramp1 : simulink/Sources/Ramp  slope=1  start=3  InitialOutput=0
  Ramp2 : simulink/Sources/Ramp  slope=1  start=3  InitialOutput=0
  Saturation : Saturate  UpperLimit=70  LowerLimit=-70
  Saturation1 : Saturate  UpperLimit=70  LowerLimit=-70
  Saturation2 : Saturate  UpperLimit=70  LowerLimit=-70
  Saturation3 : Saturate  UpperLimit=800
  Step{,2,4,6..7} (5 alike) : Step  Time=3  SampleTime=0
  Step1 : Step  SampleTime=0
  Step3 : Step  SampleTime=0
  Step5 : Step  SampleTime=0
  Sum : Sum  Inputs=|++
  Switch{,1..7} (8 alike) : Switch  Criteria=u2 > Threshold  SaturateOnIntegerOverflow=off  InputSameDT=off
  tag scope: Vdc_Load=global, Vg_aref=global, i_B=global, i_R=global, i_Y=global
  wires:
  Step/1 -> Switch/2
  Sum/1 -> Switch/1
  [Vdc_load] -> Sum/1
  [Vdc_load] -> Switch/3
  Constant/1 -> Sum/2
  Switch/1 -> Switch7/1, Saturation3/1
  [Vg_a_ref] -> Gain/1
  Gain/1 -> [Vg_aref]
  Ramp/1 -> MATLAB Function/1(u)
  Gain4/1 -> Gain1/1, Switch1/3
  Gain1/1 -> Switch1/1
  [I_R] -> Gain4/1
  Step1/1 -> Switch1/2
  Switch1/1 -> Gain5/1, Switch2/3
  Step2/1 -> Switch2/2
  Gain5/1 -> Switch2/1
  Step4/1 -> Switch4/2
  Gain6/1 -> Switch4/1
  Gain3/1 -> Gain2/1, Switch3/3
  Switch3/1 -> Gain6/1, Switch4/3
  [I_Y] -> Gain3/1
  Gain2/1 -> Switch3/1
  Ramp1/1 -> MATLAB Function1/1(u)
  Step3/1 -> Switch3/2
  Step5/1 -> Switch5/2
  Ramp2/1 -> MATLAB Function2/1(u)
  Gain7/1 -> Switch5/1
  Switch5/1 -> Gain9/1, Switch6/3
  Gain8/1 -> Gain7/1, Switch5/3
  Gain9/1 -> Switch6/1
  [I_B] -> Gain8/1
  Step6/1 -> Switch6/2
  Switch2/1 -> Saturation/1
  Saturation/1 -> [i_R]
  Switch4/1 -> Saturation2/1
  Saturation2/1 -> [i_Y]
  Switch6/1 -> Saturation1/1
  Saturation1/1 -> [i_B]
  Saturation3/1 -> Switch7/3
  Step7/1 -> Switch7/2
  Switch7/1 -> [Vdc_Load]

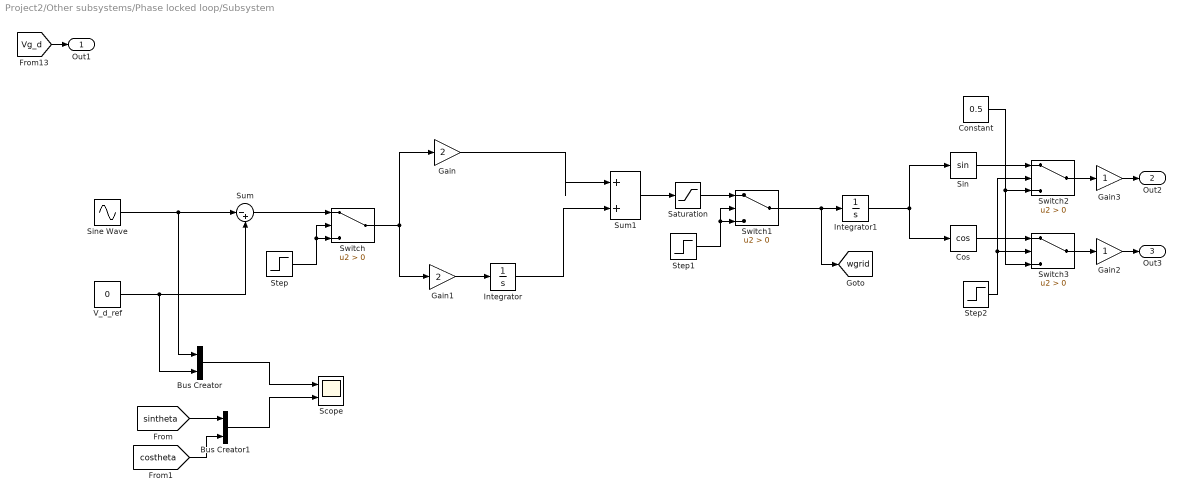
== system Project2/Other subsystems/Phase locked loop/Subsystem ==
  Bus Creator : BusCreator  Inputs=2
  Bus Creator1 : BusCreator  Inputs=2
  Constant : Constant  Value=0.5
  Cos : Trigonometry  Operator=cos
  Gain : Gain  Gain=2
  Gain1 : Gain  Gain=2
  Gain2 : Gain
  Gain3 : Gain
  Integrator : Integrator  LimitOutput=on  UpperSaturationLimit=2*pi*70  LowerSaturationLimit=-2*pi*70
  Integrator1 : Integrator
  Saturation : Saturate  UpperLimit=2*pi*70  LowerLimit=-2*pi*70
  Scope : Scope  NumInputPorts=2
  Sin : Trigonometry
  Sine Wave : Sin  Amplitude=200  Frequency=100*pi  SampleTime=0
  Step : Step  Time=0.3  SampleTime=0
  Step1 : Step  Time=0.3  SampleTime=0
  Step2 : Step  Time=0.3  SampleTime=0
  Sum : Sum  Inputs=|-+
  Sum1 : Sum  Inputs=|++
  Switch{,1..3} (4 alike) : Switch  Criteria=u2 > Threshold  SaturateOnIntegerOverflow=off  InputSameDT=off
  V_d_ref : Constant  Value=0
  Out1 : Outport
  Out2 : Outport  Port=2
  Out3 : Outport  Port=3
  tag scope: wgrid=global
  wires:
  Gain3/1 -> Out2/1
  Gain2/1 -> Out3/1
  Gain1/1 -> Integrator/1
  Sum/1 -> Switch/1
  Bus Creator1/1 -> Scope/2
  V_d_ref/1 -> Bus Creator/2, Sum/2
  Step/1 -> Switch/3, Switch/2
  Saturation/1 -> Switch1/1
  Switch3/1 -> Gain2/1
  Integrator1/1 -> Cos/1, Sin/1
  Switch/1 -> Gain1/1, Gain/1
  Sin/1 -> Switch2/1
  [sintheta] -> Bus Creator1/1
  Sum1/1 -> Saturation/1
  Step2/1 -> Switch2/2, Switch3/2
  Switch2/1 -> Gain3/1
  Sine Wave/1 -> Bus Creator/1, Sum/1
  Bus Creator/1 -> Scope/1
  Integrator/1 -> Sum1/2
  [costheta] -> Bus Creator1/2
  Step1/1 -> Switch1/3, Switch1/2
  Gain/1 -> Sum1/1
  Switch1/1 -> [wgrid], Integrator1/1
  Constant/1 -> Switch2/3, Switch3/3
  Cos/1 -> Switch3/1
  [Vg_d] -> Out1/1

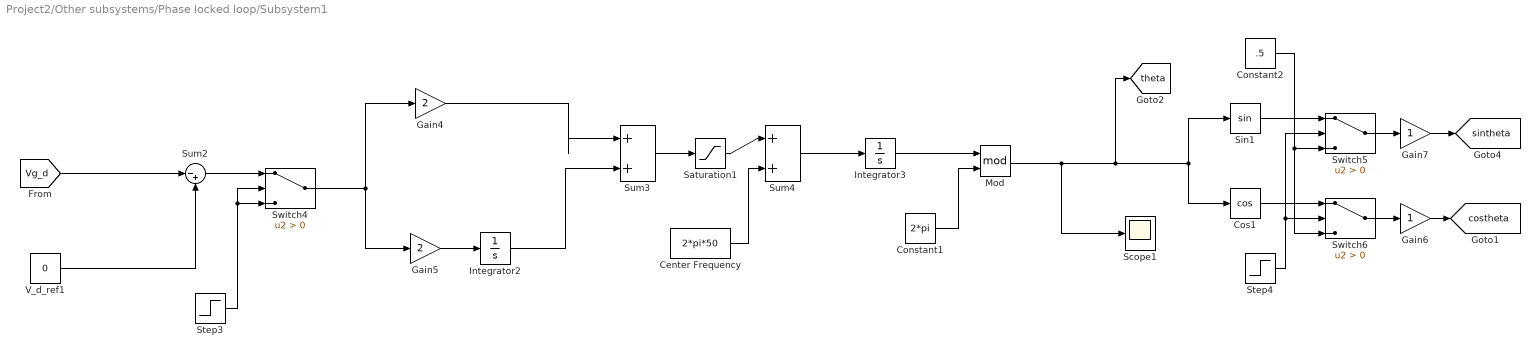
== system Project2/Other subsystems/Phase locked loop/Subsystem1 ==
  Center Frequency : Constant  Value=2*pi*50
  Constant1 : Constant  Value=2*pi
  Constant2 : Constant  Value=.5
  Cos1 : Trigonometry  Operator=cos
  Gain4 : Gain  Gain=2
  Gain5 : Gain  Gain=2
  Gain6 : Gain
  Gain7 : Gain
  Integrator2 : Integrator  LimitOutput=on  UpperSaturationLimit=2*pi*50  LowerSaturationLimit=-2*pi*50
  Integrator3 : Integrator
  Mod : Math  Operator=mod
  Saturation1 : Saturate  UpperLimit=2*pi*60  LowerLimit=-2*pi*60
  Scope1 : Scope
  Sin1 : Trigonometry
  Step3 : Step  Time=0.3  SampleTime=0
  Step4 : Step  Time=.3  SampleTime=0
  Sum2 : Sum  Inputs=|-+
  Sum3 : Sum  Inputs=|++
  Sum4 : Sum  Inputs=|++
  Switch4 : Switch  Criteria=u2 > Threshold  SaturateOnIntegerOverflow=off  InputSameDT=off
  Switch5 : Switch  Criteria=u2 > Threshold  SaturateOnIntegerOverflow=off  InputSameDT=off
  Switch6 : Switch  Criteria=u2 > Threshold  SaturateOnIntegerOverflow=off  InputSameDT=off
  V_d_ref1 : Constant  Value=0
  tag scope: costheta=global, sintheta=global, theta=global
  wires:
  Gain4/1 -> Sum3/1
  Switch6/1 -> Gain6/1
  Gain7/1 -> [sintheta]
  Switch5/1 -> Gain7/1
  Gain6/1 -> [costheta]
  Constant2/1 -> Switch5/3, Switch6/3
  Switch4/1 -> Gain4/1, Gain5/1
  Step3/1 -> Switch4/2, Switch4/3
  Sin1/1 -> Switch5/1
  Step4/1 -> Switch5/2, Switch6/2
  Cos1/1 -> Switch6/1
  V_d_ref1/1 -> Sum2/2
  Gain5/1 -> Integrator2/1
  Sum2/1 -> Switch4/1
  Constant1/1 -> Mod/2
  Mod/1 -> [theta], Sin1/1, Cos1/1, Scope1/1
  Center Frequency/1 -> Sum4/2
  Saturation1/1 -> Sum4/1
  Integrator2/1 -> Sum3/2
  Sum4/1 -> Integrator3/1
  Sum3/1 -> Saturation1/1
  Integrator3/1 -> Mod/1
  [Vg_d] -> Sum2/1

== matlab function Project2/Other subsystems/Gate sig generation/Subsystem2/MATLAB Function2 ==
  data: u input; y output
function y = fcn(u)

y = exp(-4*u);

== matlab function Project2/Other subsystems/Subsystem1/ab to dq ==
  data: a input; d output; b input; sintheta input; costheta input; q output

function [d,q] = fcn(a,b,sintheta,costheta)
    d = a*costheta + b*sintheta;
    q = -a*sintheta + b*costheta;
end

== matlab function Project2/Other subsystems/Subsystem/ab to dq (1) ==
  data: a input; d output; b input; sintheta input; costheta input; q output

function [d,q] = fcn(a,b,sintheta,costheta)
    d = a*costheta + b*sintheta;
    q = -a*sintheta + b*costheta;
end

== matlab function Project2/Other subsystems/Subsystem1/ryb to ab ==
  data: r input; y input; b input; a output; b output

function[a,b]= fcn(r,y,b)
    a= r-(b+y)/2;
    b= (y-b)*sqrt(3)/2;
end

== matlab function Project2/Other subsystems/Subsystem/ry,yb to ab ==
  data: a output; b output; ry input; yb input

function[a,b]= fcn(ry,yb)
    br= -(ry+yb);

    r= (ry-br)/3;
    b= (br-yb)/3;
    y= (yb-ry)/3;

    a= r-(y+b)/2;
    b= (y-b)*sqrt(3)/2;

end

== matlab function Project2/Other subsystems/Gate sig generation/ab to RYB ==
  data: a input; mR output; b input; mY output; mB output
function [mR,mY,mB] = fcn(a,b)
    mR=2*a/3;
    mY=-a/3+b/sqrt(3);
    mB=-a/3-b/sqrt(3);
end

== matlab function Project2/Other subsystems/Gate sig generation/dq to ab ==
  data: d input; a output; b output; q input; sintheta input; costheta input
function [a,b] =  fcn(d,q,sintheta,costheta)
    b = d*sintheta + q*costheta;
    a = d*costheta - q*sintheta;
end

== matlab function Project2/Other subsystems/V_RYB to V_Alpha-Beta/MATLAB Function ==
  data: r output; ry input; y output; yb input; b output
function [r,y,b] = fcn(ry,yb)
    br=-ry-yb;
    r=(ry-br)/3;
    y=(yb-ry)/3;
    b=(br-yb)/3;

== matlab function Project2/Other subsystems/Gate sig generation/Subsystem2/MATLAB Function ==
  data: u input; y output
function y = fcn(u)

y = exp(-4*u);

== matlab function Project2/Other subsystems/Gate sig generation/Subsystem2/MATLAB Function1 ==
  data: u input; y output
function y = fcn(u)

y = exp(-4*u);
